simulink subsystem "subrSinglePhaseMotorElectrics"  (R2024a)
settings: Solver=VariableStepAuto  StartTime=0.0  StopTime=10.0  RelTol=1e-3
model mask{RL=RL, LL=LL, KB=KB, KT=KT}
  mask prompts: RL "Resistance"; LL "Inductance"; KB "Voltage Constant"; KT "Troque Constant"
undefined symbols (not defined in the file): MOTR
settings Model: Creator=anant  LastModifiedBy=anant

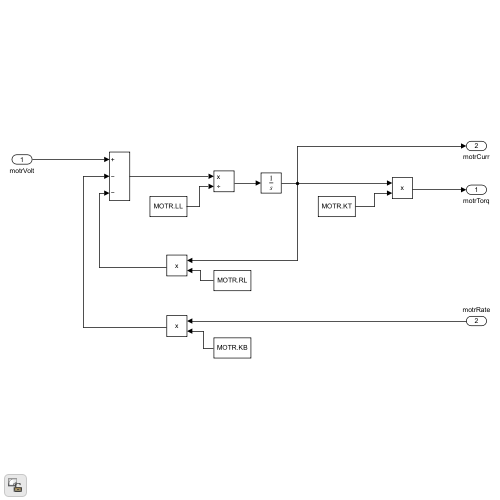
[thumbnail: Simulink's stored preview of the top-level diagram]
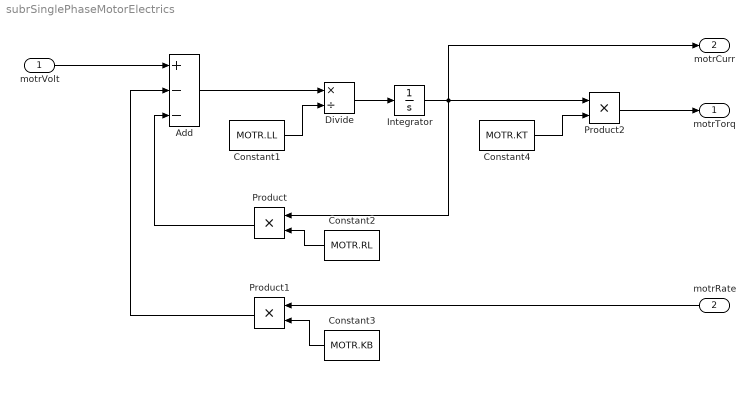
== system subrSinglePhaseMotorElectrics ==
  motrVolt : Inport
  motrRate : Inport  Port=2
  Add : Sum  Inputs=+--
  Constant1 : Constant  Value=MOTR.LL
  Constant2 : Constant  Value=MOTR.RL
  Constant3 : Constant  Value=MOTR.KB
  Constant4 : Constant  Value=MOTR.KT
  Divide : Product  Inputs=*/
  Integrator : Integrator
  Product : Product
  Product1 : Product
  Product2 : Product
  motrTorq : Outport
  motrCurr : Outport  Port=2
  wires:
  Constant3/1 -> Product1/2
  Product/1 -> Add/3
  Constant2/1 -> Product/2
  Add/1 -> Divide/1
  Constant4/1 -> Product2/2
  Integrator/1 -> Product2/1, motrCurr/1, Product/1
  Divide/1 -> Integrator/1
  Constant1/1 -> Divide/2
  Product1/1 -> Add/2
  Product2/1 -> motrTorq/1
  motrVolt/1 -> Add/1
  motrRate/1 -> Product1/1
